simulink library "library"  (R2018b)
settings: Solver=VariableStepAuto  StartTime=0.0  StopTime=10.0  RelTol=1e-3
values from neighbouring files (symbols this model uses):
  fi_param = int32(2^0)    [setup.m]
libraries: simulink x2
settings Model: Creator=hiterd  LastModifiedBy=hiterd

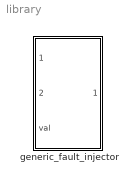
== system library ==
  generic_fault_injector : Subsystem

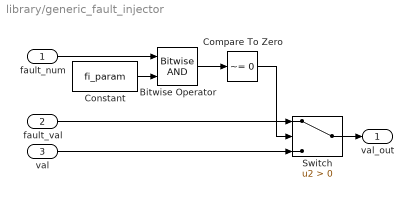
== system library/generic_fault_injector ==
  fault_num : Inport
  fault_val : Inport  Port=2
  val : Inport  Port=3
  Bitwise Operator : simulink/Logic and Bit Operations/Bitwise Operator  logicop=AND  UseBitMask=off  NumInputPorts=2  BitMask=bin2dec('fi_param')  BitMaskRealWorld=Stored Integer
  Compare To Zero : simulink/Logic and Bit Operations/Compare To Zero  relop=~=  OutDataTypeStr=boolean
  Constant : Constant  Value=fi_param  SampleTime=-1
  Switch : Switch  Criteria=u2 > Threshold
  val_out : Outport
  wires:
  fault_num/1 -> Bitwise Operator/1
  Compare To Zero/1 -> Switch/2
  fault_val/1 -> Switch/1
  Bitwise Operator/1 -> Compare To Zero/1
  val/1 -> Switch/3
  Switch/1 -> val_out/1
  Constant/1 -> Bitwise Operator/2
